simulink model "C20259_DiegoAlfaro_G01"  (R2023b)
settings: Solver=VariableStepAuto  StartTime=0.0  StopTime=4000  FixedStep=1e-3  RelTol=1e-3
undefined symbols (not defined in the file): A, deltad, deltau, g, H0, K1, K2, Kt, Kvc, Kvs, rho, steptimed, steptimeu, T, u0, Xvs0
settings Model: Creator=daas0  LastModifiedBy=daas0

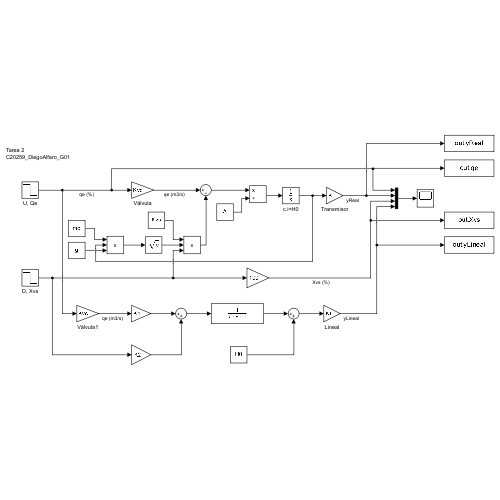
[thumbnail: Simulink's stored preview of the top-level diagram]
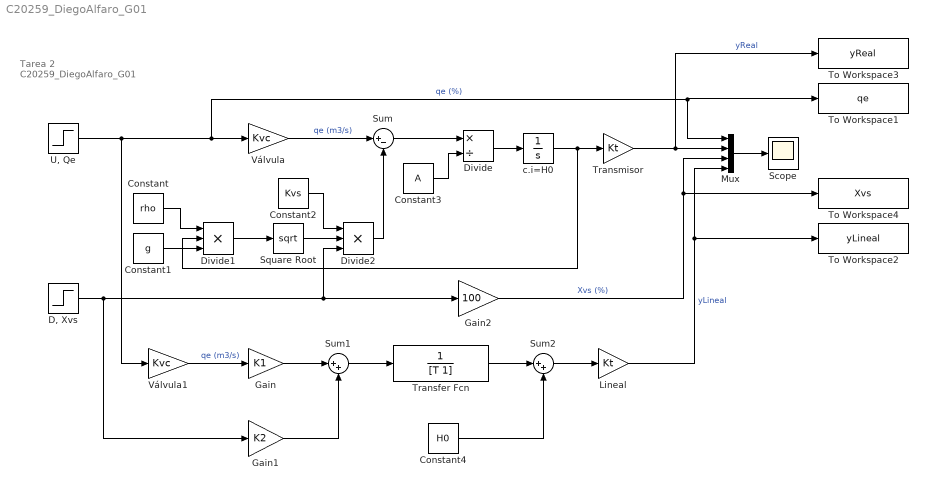
== system C20259_DiegoAlfaro_G01 ==
  note: Tarea 2
      | C20259_DiegoAlfaro_G01
  Constant : Constant  Value=rho
  Constant1 : Constant  Value=g
  Constant2 : Constant  Value=Kvs
  Constant3 : Constant  Value=A
  Constant4 : Constant  Value=H0
  "D, Xvs" : Step  Time=steptimed  Before=Xvs0  After=deltad  SampleTime=0
  Divide : Product  Inputs=*/
  Divide1 : Product  Inputs=***
  Divide2 : Product  Inputs=***
  Gain : Gain  Gain=K1
  Gain1 : Gain  Gain=K2
  Gain2 : Gain  Gain=100
  Lineal : Gain  Gain=Kt
  Mux : Mux
  Scope : Scope
  Square Root : Sqrt
  Sum : Sum  Inputs=|+-
  Sum1 : Sum  Inputs=|++
  Sum2 : Sum  Inputs=|++
  To Workspace1 : ToWorkspace  VariableName=qe  SaveFormat=Timeseries  SampleTime=-1
  To Workspace2 : ToWorkspace  VariableName=yLineal  SaveFormat=Timeseries  SampleTime=-1
  To Workspace3 : ToWorkspace  VariableName=yReal  SaveFormat=Timeseries  SampleTime=-1
  To Workspace4 : ToWorkspace  VariableName=Xvs  SaveFormat=Timeseries  SampleTime=-1
  Transfer Fcn : TransferFcn  Denominator=[T 1]
  Transmisor : Gain  Gain=Kt
  "U, Qe" : Step  Time=steptimeu  Before=u0  After=deltau  SampleTime=0
  Válvula : Gain  Gain=Kvc
  Válvula1 : Gain  Gain=Kvc
  c.i=H0 : Integrator  InitialCondition=H0
  wires:
  "U, Qe"/1 -> Válvula1/1, Válvula/1, Mux/1, To Workspace1/1  "qe (%)"
  Constant/1 -> Divide1/1
  Constant1/1 -> Divide1/3
  Divide1/1 -> Square Root/1
  Square Root/1 -> Divide2/2
  Constant2/1 -> Divide2/1
  Válvula/1 -> Sum/1  "qe (m3/s)"
  Divide2/1 -> Sum/2
  Sum/1 -> Divide/1
  Constant3/1 -> Divide/2
  Divide/1 -> c.i=H0/1
  c.i=H0/1 -> Divide1/2, Transmisor/1
  "D, Xvs"/1 -> Gain1/1, Divide2/3, Gain2/1
  Transmisor/1 -> Mux/2, To Workspace3/1  "yReal"
  Gain2/1 -> Mux/3, To Workspace4/1  "Xvs (%)"
  Mux/1 -> Scope/1
  Válvula1/1 -> Gain/1  "qe (m3/s)"
  Gain/1 -> Sum1/1
  Gain1/1 -> Sum1/2
  Sum1/1 -> Transfer Fcn/1
  Transfer Fcn/1 -> Sum2/1
  Constant4/1 -> Sum2/2
  Sum2/1 -> Lineal/1
  Lineal/1 -> To Workspace2/1, Mux/4  "yLineal"
